simulink model "EthernetDrone"  (Simulink 8.5)
settings: Solver=ode45  StartTime=0.0  StopTime=300  RelTol=abstol/10  AbsTol=abstol
undefined symbols (not defined in the file or in its folder): A, a_noise_seed, a_noise_var, Cd, enu2ecef, g, GPS_DT, h_noise_seed, h_noise_var, I, I_motor, IMU_DT, m, mag_bias, MAG_DT, mag_noise_seed, mag_noise_var, MaxPropRate, MaxPwmWidth, mean_a_bias, mean_w_bias, MinPwmWidth, q0, r0, r1, r2, r3, r4, r_gps, RateToForce, Re, rho, v0, v_noise_seed, v_noise_var, w0, w_noise_seed, w_noise_var
libraries: simulink x7, instrumentlib x4
settings Model: Creator=Mike  LastModifiedBy=Walker  CovSFcnEnable=off
settings SolverCC: ZeroCrossControl=DisableAll
settings DebuggingCC: SolverPrmCheckMsg=warning  FcnCallInpInsideContextMsg=UseLocalSettings

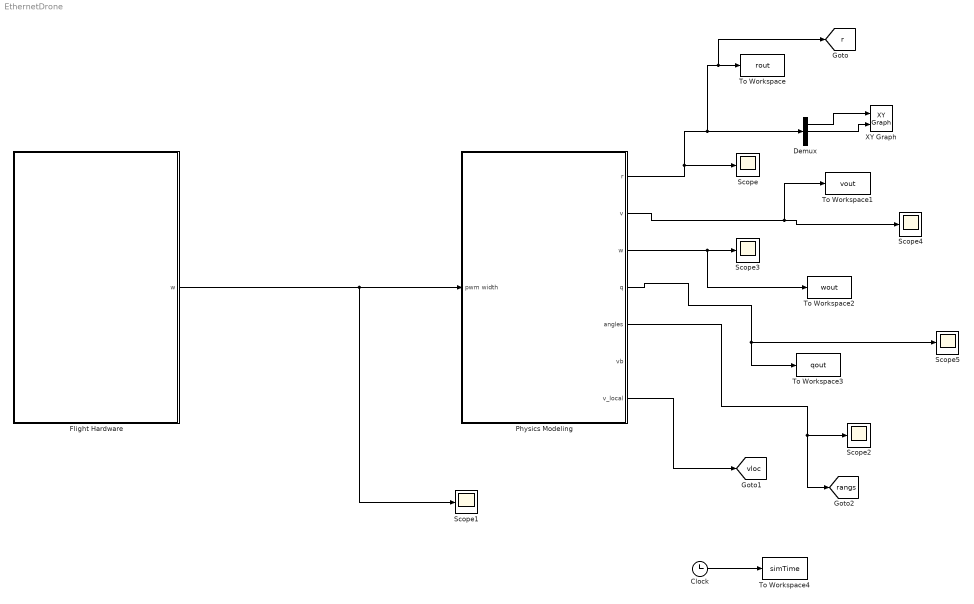
== system EthernetDrone ==
  Clock : Clock
  Demux : Demux  Outputs=3
  Flight Hardware : Subsystem
  Physics Modeling : Subsystem
  Scope{,1..5} (6 alike) : Scope
      Scope settings: TimeRange=100  YMin=4  YMax=17
      Scope1 settings: TimeRange=10  YMin=1.368  YMax=1.3696
      Scope2 settings: TimeRange=300  YMin=-4.5  YMax=4.5  SaveName=ScopeData5
      Scope3 settings: TimeRange=30  YMin=-0.05  YMax=0.05  SaveName=ScopeData13
      Scope4 settings: TimeRange=100  YMin=-4  YMax=8  SaveName=ScopeData38
      Scope5 settings: TimeRange=100  YMin=-0.2  YMax=1  SaveName=ScopeData96
  To Workspace : ToWorkspace  VariableName=rout  SampleTime=IMU_DT
  To Workspace1 : ToWorkspace  VariableName=vout  SampleTime=IMU_DT
  To Workspace2 : ToWorkspace  VariableName=wout  SampleTime=IMU_DT
  To Workspace3 : ToWorkspace  VariableName=qout  SampleTime=IMU_DT
  To Workspace4 : ToWorkspace  VariableName=simTime  SampleTime=IMU_DT
  XY Graph : simulink/Sinks/XY Graph  xmin=-20  xmax=20  ymin=-20  ymax=20  st=1
  tag scope: r=global, rangs=global, vloc=global
  wires:
  Flight Hardware/1(w) -> Physics Modeling/1("pwm width "), Scope1/1
  Physics Modeling/1(r) -> Demux/1, To Workspace/1, [r], Scope/1
  Physics Modeling/5(angles) -> Scope2/1, [rangs]
  Physics Modeling/3(w) -> Scope3/1, To Workspace2/1
  Physics Modeling/2(v) -> Scope4/1, To Workspace1/1
  Demux/1 -> XY Graph/1
  Demux/2 -> XY Graph/2
  Physics Modeling/4(q) -> To Workspace3/1, Scope5/1
  Physics Modeling/7(v_local) -> [vloc]
  Clock/1 -> To Workspace4/1

== system EthernetDrone/Flight Hardware ==
  Sensor Model : Subsystem
  Subsystem : Subsystem
  Subsystem1 : Subsystem
  Subsystem2 : Subsystem
  Subsystem3 : Subsystem
  w : Outport
  wires:
  Sensor Model/2(w_b) -> Subsystem/2(win)
  Sensor Model/1(a_b) -> Subsystem/1(ain)
  Sensor Model/3(h) -> Subsystem1/1(gps)
  Sensor Model/4(mag) -> Subsystem2/1(mag)
  Subsystem3/1(w) -> w/1

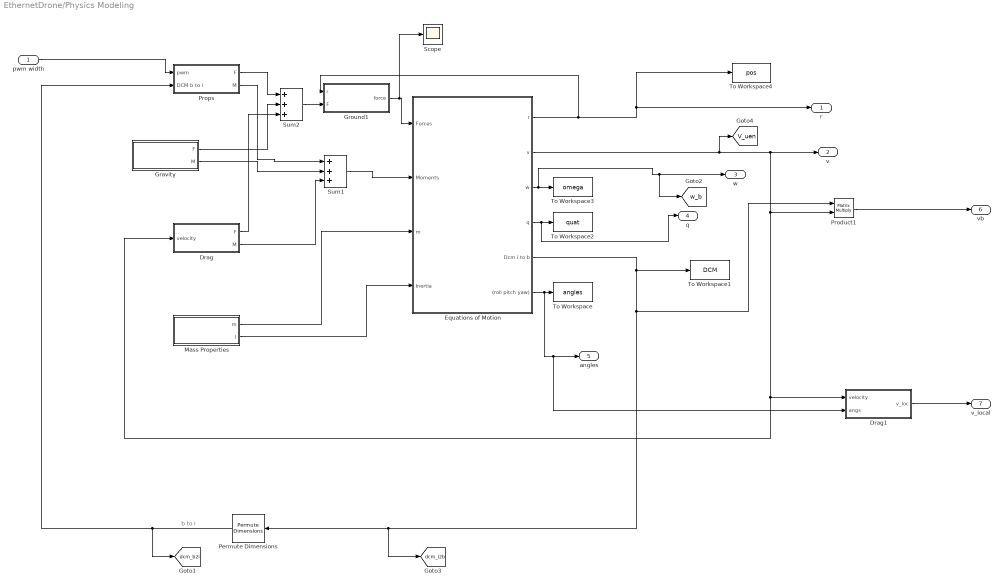
== system EthernetDrone/Physics Modeling ==
  note: b to i
  "pwm width " : Inport
  Drag : Subsystem
  Drag1 : Subsystem
  Equations of Motion : Subsystem
  Gravity : Subsystem
  Ground1 : Subsystem
  Mass Properties : Subsystem
  Permute Dimensions : PermuteDimensions
  Product1 : Product  Multiplication=Matrix(*)  RndMeth=Zero
  Props : Subsystem
  Scope : Scope
      settings: TimeRange=5.350553505535055  YMin=-4  SaveName=ScopeData58
  Sum1 : Sum  Inputs=+++
  Sum2 : Sum  Inputs=+++
  To Workspace : ToWorkspace  VariableName=angles  SampleTime=-1
  To Workspace1 : ToWorkspace  VariableName=DCM  SampleTime=-1
  To Workspace2 : ToWorkspace  VariableName=quat  SampleTime=-1
  To Workspace3 : ToWorkspace  VariableName=omega  SampleTime=-1
  To Workspace4 : ToWorkspace  VariableName=pos  SampleTime=-1
  r : Outport
  v : Outport  Port=2
  w : Outport  Port=3
  q : Outport  Port=4
  angles : Outport  Port=5
  vb : Outport  Port=6
  v_local : Outport  Port=7
  tag scope: V_uen=global, dcm_b2i=global, dcm_i2b=global, w_b=global
  wires:
  Props/1(F) -> Sum2/1
  Gravity/1(F) -> Sum2/2
  Drag/1(F) -> Sum2/3
  Props/2(M) -> Sum1/1
  Gravity/2(M) -> Sum1/2
  Drag/2(M) -> Sum1/3
  Sum1/1 -> Equations of Motion/2(Moments)
  Mass Properties/1(m) -> Equations of Motion/3(m)
  Mass Properties/2(I) -> Equations of Motion/4(Inertia)
  "pwm width "/1 -> Props/1(pwm)
  Equations of Motion/2(v) -> Drag/1(velocity), Drag1/1(velocity), Product1/2, v/1, [V_uen]
  Equations of Motion/1(r) -> Ground1/1(r), To Workspace4/1, r/1
  Equations of Motion/6((roll pitch yaw)) -> To Workspace/1, angles/1, Drag1/2(angs)
  Equations of Motion/5(Dcm i to b) -> To Workspace1/1, Product1/1, Permute Dimensions/1, [dcm_i2b]
  Equations of Motion/4(q) -> To Workspace2/1, q/1
  Equations of Motion/3(w) -> To Workspace3/1, w/1, [w_b]
  Permute Dimensions/1 -> [dcm_b2i], Props/2("DCM b to i ")
  Product1/1 -> vb/1
  Drag1/1(v_loc) -> v_local/1
  Ground1/1(force) -> Scope/1, Equations of Motion/1(Forces)
  Sum2/1 -> Ground1/2(F)

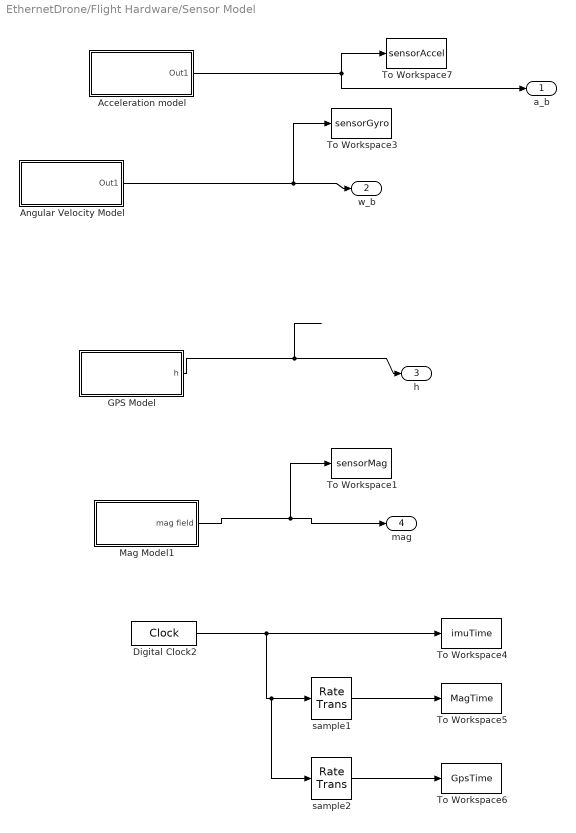
== system EthernetDrone/Flight Hardware/Sensor Model ==
  Acceleration model : Subsystem
  Angular Velocity Model : Subsystem
  Digital Clock2 : DigitalClock  SampleTime=IMU_DT
  GPS Model : Subsystem
  Mag Model1 : Subsystem
  To Workspace1 : ToWorkspace  VariableName=sensorMag  SampleTime=-1
  To Workspace3 : ToWorkspace  VariableName=sensorGyro  SampleTime=-1
  To Workspace4 : ToWorkspace  VariableName=imuTime  SampleTime=-1
  To Workspace5 : ToWorkspace  VariableName=MagTime  SampleTime=-1
  To Workspace6 : ToWorkspace  VariableName=GpsTime  SampleTime=-1
  To Workspace7 : ToWorkspace  VariableName=sensorAccel  SampleTime=-1
  sample1 : RateTransition  OutPortSampleTime=MAG_DT
  sample2 : RateTransition  OutPortSampleTime=GPS_DT
  a_b : Outport
  w_b : Outport  Port=2
  h : Outport  Port=3
  mag : Outport  Port=4
  wires:
  Acceleration model/1(Out1) -> a_b/1, To Workspace7/1
  Angular Velocity Model/1(Out1) -> To Workspace3/1, w_b/1
  GPS Model/1(h) -> h/1
  Mag Model1/1(mag field) -> To Workspace1/1, mag/1
  Digital Clock2/1 -> To Workspace4/1, sample1/1, sample2/1
  sample1/1 -> To Workspace5/1
  sample2/1 -> To Workspace6/1

== system EthernetDrone/Flight Hardware/Subsystem ==
  ain : Inport
  win : Inport  Port=2
  Digital Clock : DigitalClock  SampleTime=IMU_DT
  Mux : Mux  Inputs=3
  UDP Send : instrumentlib/UDP Send  Host=127.0.0.1  Port=8000  LocalPort=-1  EnableBlockingMode=on  ByteOrder=LittleEndian
  wires:
  ain/1 -> Mux/1
  win/1 -> Mux/2
  Digital Clock/1 -> Mux/3
  Mux/1 -> UDP Send/1

== system EthernetDrone/Flight Hardware/Subsystem1 ==
  gps : Inport
  Digital Clock : DigitalClock  SampleTime=GPS_DT
  Mux : Mux  Inputs=2
  UDP Send : instrumentlib/UDP Send  Host=127.0.0.1  Port=8100  LocalPort=-1  EnableBlockingMode=on  ByteOrder=LittleEndian
  wires:
  gps/1 -> Mux/1
  Digital Clock/1 -> Mux/2
  Mux/1 -> UDP Send/1

== system EthernetDrone/Flight Hardware/Subsystem2 ==
  mag : Inport
  Digital Clock : DigitalClock  SampleTime=MAG_DT
  Mux : Mux  Inputs=2
  UDP Send : instrumentlib/UDP Send  Host=127.0.0.1  Port=8200  LocalPort=-1  EnableBlockingMode=on  ByteOrder=LittleEndian
  wires:
  mag/1 -> Mux/1
  Digital Clock/1 -> Mux/2
  Mux/1 -> UDP Send/1

== system EthernetDrone/Flight Hardware/Subsystem3 ==
  Data Type Conversion : DataTypeConversion  OutDataTypeStr=double  SampleTime=IMU_DT
  UDP Receive : instrumentlib/UDP Receive  Host=127.0.0.1  Port=8300  LocalPort=8300  DataSize=4  EnableBlockingMode=on  Timeout=10  SampleTime=-1  DataType=double  ByteOrder=LittleEndian
  w : Outport
  wires:
  UDP Receive/1 -> Data Type Conversion/1
  Data Type Conversion/1 -> w/1

== system EthernetDrone/Physics Modeling/Drag ==
  velocity : Inport
  Abs : Abs
  Constant : Constant  Value=rho*Cd*A
  Gain : Gain  Gain=-0.5
  Product : Product  Inputs=***  RndMeth=Zero
  Scope : Scope
      settings: TimeRange=80  SaveName=ScopeData54
  assume cp = cm : Constant  Value=0
  F : Outport
  M : Outport  Port=2
  tag scope: faero_i=global
  wires:
  velocity/1 -> Abs/1, Gain/1
  Gain/1 -> Product/2
  Abs/1 -> Product/1
  Constant/1 -> Product/3
  assume cp = cm/1 -> M/1
  Product/1 -> F/1, [faero_i], Scope/1

== system EthernetDrone/Physics Modeling/Drag1 ==
  velocity : Inport
  angs : Inport  Port=2
  Embedded MATLAB Function : MATLAB Function  TreatAsAtomicUnit=on
  Product : Product  Multiplication=Matrix(*)  RndMeth=Zero
  v_loc : Outport
  wires:
  velocity/1 -> Product/2
  Product/1 -> v_loc/1
  angs/1 -> Embedded MATLAB Function/1(u)
  Embedded MATLAB Function/1(y) -> Product/1

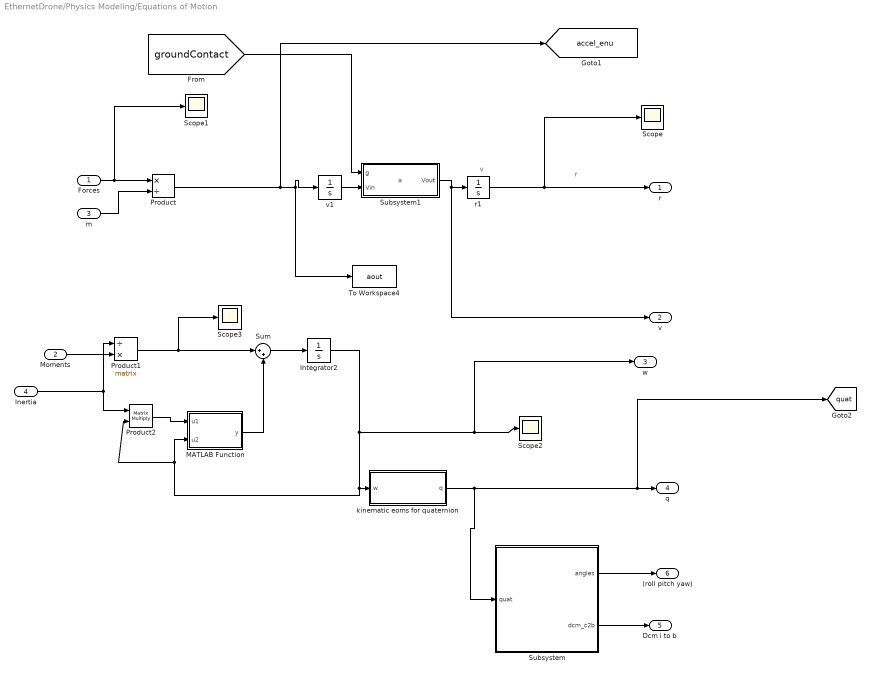
== system EthernetDrone/Physics Modeling/Equations of Motion ==
  note: a
  note: v
  note: r
  Forces : Inport
  Moments : Inport  Port=2
  m : Inport  Port=3
  Inertia : Inport  Port=4
  Integrator2 : Integrator  InitialCondition=w0  AbsoluteTolerance=abstol
  MATLAB Function : MATLAB Function  TreatAsAtomicUnit=on
  Product : Product  Inputs=*/  RndMeth=Zero
  Product1 : Product  Inputs=/*  Multiplication=Matrix(*)  RndMeth=Zero
  Product2 : Product  Inputs=**  Multiplication=Matrix(*)  RndMeth=Zero
  Scope{,1..3} (4 alike) : Scope
      Scope settings: SaveName=ScopeData55
      Scope1 settings: TimeRange=100  SaveName=ScopeData56
      Scope2 settings: TimeRange=50  YMin=-2000  YMax=0  SaveName=ScopeData14
      Scope3 settings: TimeRange=50  YMin=-2000  YMax=0  SaveName=ScopeData37
  Subsystem : Subsystem
  Subsystem1 : Subsystem
  Sum : Sum  Inputs=|++
  To Workspace4 : ToWorkspace  VariableName=aout  SampleTime=-1
  kinematic eoms for quaternion : Subsystem
  r1 : Integrator  InitialCondition=r0  AbsoluteTolerance=abstol
  v1 : Integrator  InitialCondition=v0  AbsoluteTolerance=abstol
  r : Outport
  v : Outport  Port=2
  w : Outport  Port=3
  q : Outport  Port=4
  Dcm i to b : Outport  Port=5
  (roll pitch yaw) : Outport  Port=6
  tag scope: accel_enu=global, quat=global
  wires:
  r1/1 -> Scope/1, r/1
  Forces/1 -> Product/1, Scope1/1
  m/1 -> Product/2
  kinematic eoms for quaternion/1(q) -> Subsystem/1(quat), q/1, [quat]
  Subsystem/2(dcm_c2b) -> Dcm i to b/1
  Subsystem/1(angles) -> (roll pitch yaw)/1
  Inertia/1 -> Product1/1, Product2/1
  Moments/1 -> Product1/2
  Integrator2/1 -> Scope2/1, w/1, kinematic eoms for quaternion/1(w), MATLAB Function/2(u2), Product2/2
  Product2/1 -> MATLAB Function/1(u1)
  Sum/1 -> Integrator2/1
  Product1/1 -> Sum/1, Scope3/1
  MATLAB Function/1(y) -> Sum/2
  Product/1 -> [accel_enu], v1/1, To Workspace4/1
  Subsystem1/1(Vout) -> v/1, r1/1
  v1/1 -> Subsystem1/2(Vin)
  [groundContact] -> Subsystem1/1(g)

== system EthernetDrone/Physics Modeling/Gravity ==
  Ground1 : Subsystem
  No horizontal : Gain  Gain=m
  Scope : Scope
      settings: SaveName=ScopeData57
  cg=cm in this problem : Constant  Value=0
  mg : Constant  Value=[0;0; -m*g ]
  F : Outport
  M : Outport  Port=2
  wires:
  cg=cm in this problem/1 -> M/1
  mg/1 -> F/1, Scope/1
  Ground1/1(accel) -> No horizontal/1

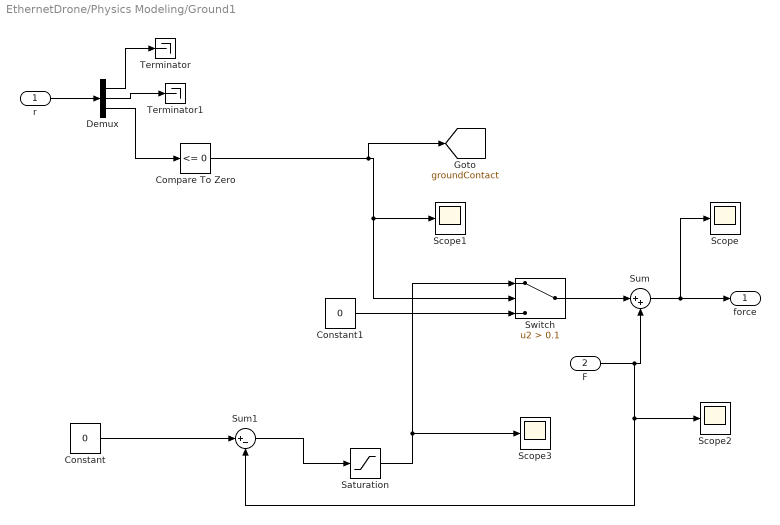
== system EthernetDrone/Physics Modeling/Ground1 ==
  r : Inport
  F : Inport  Port=2
  Compare To Zero : simulink/Logic and Bit Operations/Compare To Zero  relop=<=  OutDataTypeStr=boolean  ZeroCross=off
  Constant : Constant  Value=0
  Constant1 : Constant  Value=0
  Demux : Demux  Outputs=3
  Saturation : Saturate  UpperLimit=inf  LowerLimit=0
  Scope{,1..3} (4 alike) : Scope
      Scope settings: YMin=-10  YMax=10  SaveName=ScopeData88
      Scope1 settings: TimeRange=20  YMin=0.95  YMax=1.05  SaveName=ScopeData51
      Scope2 settings: YMin=-10  YMax=0  SaveName=ScopeData127
      Scope3 settings: YMin=9.5  YMax=20  SaveName=ScopeData128
  Sum : Sum  Inputs=|++
  Sum1 : Sum  Inputs=|+-
  Switch : Switch  Criteria=u2 > Threshold  Threshold=0.1
  Terminator : Terminator
  Terminator1 : Terminator
  force : Outport
  tag scope: groundContact=global
  wires:
  r/1 -> Demux/1
  Demux/1 -> Terminator/1
  Demux/2 -> Terminator1/1
  Demux/3 -> Compare To Zero/1
  Compare To Zero/1 -> [groundContact], Scope1/1, Switch/2
  Saturation/1 -> Switch/1, Scope3/1
  Switch/1 -> Sum/1
  Sum/1 -> Scope/1, force/1
  F/1 -> Scope2/1, Sum1/2, Sum/2
  Constant/1 -> Sum1/1
  Sum1/1 -> Saturation/1
  Constant1/1 -> Switch/3

== system EthernetDrone/Physics Modeling/Mass Properties ==
  Constant : Constant  Value=m
  a : Constant  Value=I
  m : Outport
  I : Outport  Port=2
  tag scope: mass=global
  wires:
  a/1 -> I/1
  Constant/1 -> m/1, [mass]

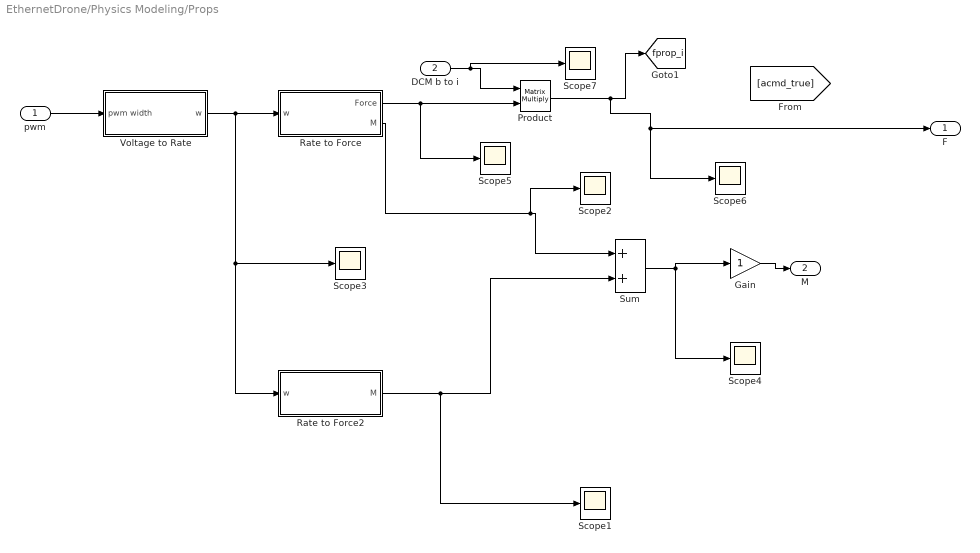
== system EthernetDrone/Physics Modeling/Props ==
  pwm : Inport
  "DCM b to i " : Inport  Port=2
  Gain : Gain
  Product : Product  Multiplication=Matrix(*)  OutDataTypeStr=Inherit: Inherit via back propagation  RndMeth=Nearest
  Rate to Force : Subsystem
  Rate to Force2 : Subsystem
  Scope{1..7} (7 alike) : Scope
      Scope1 settings: TimeRange=50  YMin=0  YMax=200  SaveName=ScopeData2
      Scope2 settings: YMin=-1  YMax=1  SaveName=ScopeData3
      Scope3 settings: TimeRange=50  YMin=-0.2  YMax=0.85  SaveName=ScopeData4
      Scope4 settings: TimeRange=6.110074626865668  YMin=-3.63961038961039e-009  YMax=-3.405844155844153e-009  SaveName=ScopeData11
      Scope5 settings: TimeRange=50  YMin=0  YMax=4e+14  SaveName=ScopeData9
      Scope6 settings: TimeRange=50  YMin=0  YMax=40  SaveName=ScopeData59
      Scope7 settings: TimeRange=0.2158273381295004  YMin=-1  YMax=1  SaveName=ScopeData62
  Sum : Sum
  Voltage to Rate : Subsystem
  F : Outport
  M : Outport  Port=2
  tag scope: fprop_i=global
  wires:
  pwm/1 -> Voltage to Rate/1(pwm width)
  Voltage to Rate/1(w) -> Rate to Force/1(w), Rate to Force2/1(w), Scope3/1
  Sum/1 -> Scope4/1, Gain/1
  Rate to Force/2(M) -> Sum/1, Scope2/1
  Rate to Force2/1(M) -> Sum/2, Scope1/1
  Product/1 -> [fprop_i], Scope6/1, F/1
  "DCM b to i "/1 -> Product/1, Scope7/1
  Rate to Force/1(Force) -> Product/2, Scope5/1
  Gain/1 -> M/1

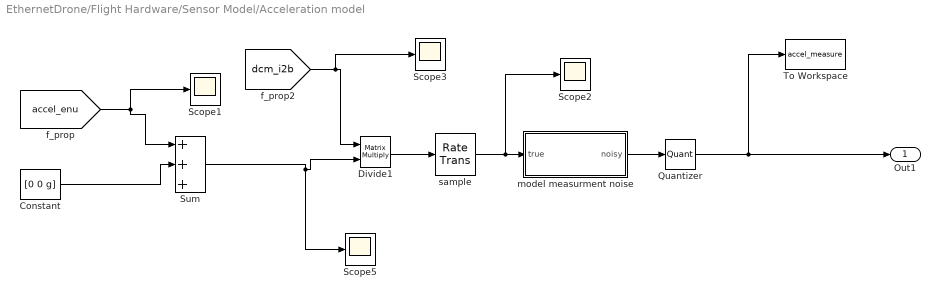
== system EthernetDrone/Flight Hardware/Sensor Model/Acceleration model ==
  Constant : Constant  Value=[0 0 g]
  Divide1 : Product  Inputs=**  Multiplication=Matrix(*)
  Quantizer : Quantizer  QuantizationInterval=AccelQuant
  Scope{1..3,5} (4 alike) : Scope
      Scope1 settings: TimeRange=30  YMin=-50  YMax=50  SaveName=ScopeData46
      Scope2 settings: TimeRange=35  YMin=-2.5  YMax=40  SaveName=ScopeData47
      Scope3 settings: TimeRange=35  YMin=0  YMax=1  SaveName=ScopeData100
      Scope5 settings: TimeRange=49.99000000000001  YMin=9.763194444444443  YMax=9.821527777777776  SaveName=ScopeData101
  Sum : Sum  Inputs=+++
  To Workspace : ToWorkspace  VariableName=accel_measure  SampleTime=-1
  model measurment noise : Subsystem
  sample : RateTransition  X0=[0 0 g]  OutPortSampleTime=IMU_DT
  Out1 : Outport
  wires:
  Constant/1 -> Sum/2
  [accel_enu] -> Sum/1, Scope1/1
  sample/1 -> model measurment noise/1("true "), Scope2/1
  Divide1/1 -> sample/1
  Sum/1 -> Divide1/2, Scope5/1
  [dcm_i2b] -> Divide1/1, Scope3/1
  model measurment noise/1(noisy) -> Quantizer/1
  Quantizer/1 -> To Workspace/1, Out1/1

== system EthernetDrone/Flight Hardware/Sensor Model/Angular Velocity Model ==
  Product : Product  Multiplication=Matrix(*)  RndMeth=Zero
  Quantizer : Quantizer  QuantizationInterval=GyroQuant
  Scope : Scope
      settings: TimeRange=30  YMin=-0.06  YMax=0.08  SaveName=ScopeData61
  Sum : Sum  Inputs=|++
  To Workspace1 : ToWorkspace  VariableName=omega_measure  SampleTime=-1
  earth rot rate (rads/sec)--assume at lat,log h (0,0,0) : Constant  Value=[0;0;0.00007272205]
  model measurment noise : Subsystem
  sample : RateTransition  OutPortSampleTime=IMU_DT
  Out1 : Outport
  wires:
  sample/1 -> model measurment noise/1("true ")
  earth rot rate (rads/sec)--assume at lat,log h (0,0,0)/1 -> Product/2
  [dcm_i2b] -> Product/1
  Product/1 -> ?
  [w_b] -> Sum/1
  Sum/1 -> sample/1
  model measurment noise/1(noisy) -> Quantizer/1
  Quantizer/1 -> To Workspace1/1, Scope/1, Out1/1

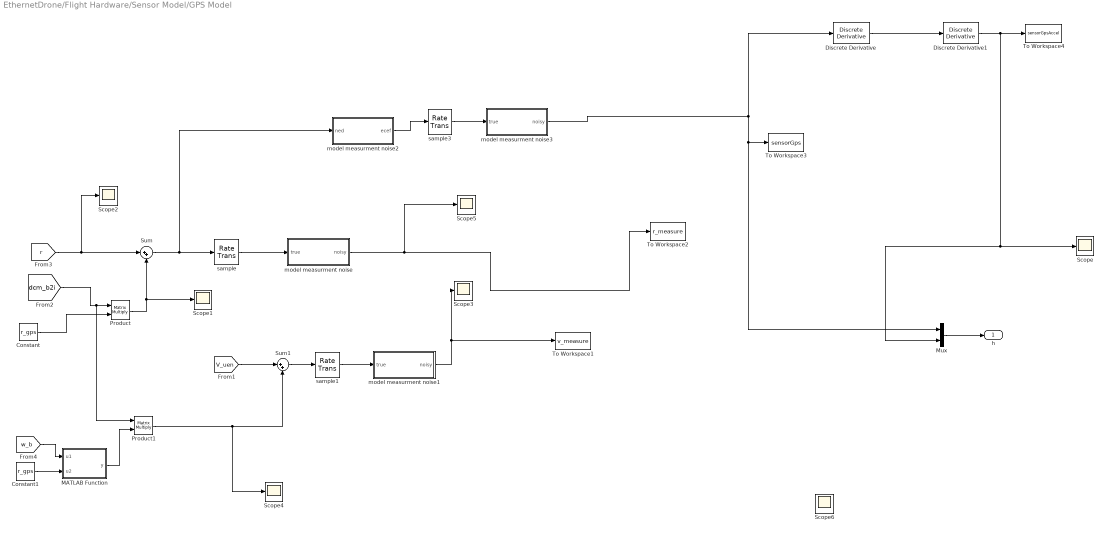
== system EthernetDrone/Flight Hardware/Sensor Model/GPS Model ==
  Constant : Constant  Value=r_gps
  Constant1 : Constant  Value=r_gps
  Discrete Derivative : simulink/Discrete/Discrete Derivative  gainval=1  ICPrevScaledInput=0.0  InputProcessing=Inherited  OutMin=[]  OutMax=[]  OutDataType=fixdt(1, 16)  OutScaling=2^-10  DoSatur=off
  Discrete Derivative1 : simulink/Discrete/Discrete Derivative  gainval=1.0  ICPrevScaledInput=0  InputProcessing=Inherited  OutMin=[]  OutMax=[]  OutDataType=fixdt(1, 16)  OutScaling=2^-10  DoSatur=off
  MATLAB Function : MATLAB Function  TreatAsAtomicUnit=on
  Mux : Mux  Inputs=2
  Product : Product  Multiplication=Matrix(*)  RndMeth=Zero
  Product1 : Product  Multiplication=Matrix(*)  RndMeth=Zero
  Scope{,1..6} (7 alike) : Scope
      Scope settings: SaveName=ScopeData49
      Scope1 settings: TimeRange=30  YMin=-1  YMax=1  SaveName=ScopeData98
      Scope2 settings: TimeRange=30  YMin=1  YMax=5.25  SaveName=ScopeData97
      Scope3 settings: TimeRange=30  YMin=-0.075  YMax=0.2  SaveName=ScopeData103
      Scope4 settings: TimeRange=30  YMin=-0.35  YMax=0.125  SaveName=ScopeData104
      Scope5 settings: TimeRange=30  YMin=3.5  YMax=11  SaveName=ScopeData94
      Scope6 settings: TimeRange=10  YMin=0.95  YMax=1.05  SaveName=ScopeData102
  Sum : Sum  Inputs=|++
  Sum1 : Sum  Inputs=|++
  To Workspace1 : ToWorkspace  VariableName=v_measure  SampleTime=GPS_DT
  To Workspace2 : ToWorkspace  VariableName=r_measure  SampleTime=IMU_DT
  To Workspace3 : ToWorkspace  VariableName=sensorGps  SampleTime=-1
  To Workspace4 : ToWorkspace  VariableName=sensorGpsAccel  SampleTime=IMU_DT
  model measurment noise : Subsystem
  model measurment noise1 : Subsystem
  model measurment noise2 : Subsystem
  model measurment noise3 : Subsystem
  sample : RateTransition  OutPortSampleTime=GPS_DT
  sample1 : RateTransition  OutPortSampleTime=GPS_DT
  sample3 : RateTransition  OutPortSampleTime=GPS_DT
  h : Outport  OutDataTypeStr=double
  wires:
  sample/1 -> model measurment noise/1("true ")
  sample1/1 -> model measurment noise1/1("true ")
  model measurment noise1/1(noisy) -> Scope3/1, To Workspace1/1
  Constant/1 -> Product/2
  [dcm_b2i] -> Product/1, Product1/1
  Sum/1 -> model measurment noise2/1("ned "), sample/1
  Product/1 -> Sum/2, Scope1/1
  [r] -> Sum/1, Scope2/1
  Sum1/1 -> sample1/1
  [V_uen] -> Sum1/1
  Constant1/1 -> MATLAB Function/2(u2)
  [w_b] -> MATLAB Function/1(u1)
  Product1/1 -> Sum1/2, Scope4/1
  MATLAB Function/1(y) -> Product1/2
  ? -> ?
  model measurment noise2/1(ecef) -> sample3/1
  sample3/1 -> model measurment noise3/1("true ")
  model measurment noise3/1(noisy) -> Discrete Derivative/1, To Workspace3/1, Mux/1
  model measurment noise/1(noisy) -> Scope5/1, To Workspace2/1
  Discrete Derivative/1 -> Discrete Derivative1/1
  Discrete Derivative1/1 -> Scope/1, Mux/2, To Workspace4/1
  Mux/1 -> h/1

== system EthernetDrone/Flight Hardware/Sensor Model/Mag Model1 ==
  Embedded MATLAB Function : MATLAB Function  TreatAsAtomicUnit=on
  Product : Product  Multiplication=Matrix(*)  RndMeth=Zero
  Scope4 : Scope
      settings: TimeRange=300  YMin=-0.8  YMax=0.05  SaveName=ScopeData108
  To Workspace3 : ToWorkspace  VariableName=mag_measure  SampleTime=MAG_DT
  model measurment noise1 : Subsystem
  sample1 : RateTransition  OutPortSampleTime=MAG_DT
  mag field : Outport  OutDataTypeStr=double
  wires:
  sample1/1 -> model measurment noise1/1("true ")
  Embedded MATLAB Function/1(Mhat) -> Product/2
  [dcm_i2b] -> Product/1
  model measurment noise1/1(noisy) -> Scope4/1, mag field/1, To Workspace3/1
  Product/1 -> sample1/1

== system EthernetDrone/Physics Modeling/Equations of Motion/Subsystem ==
  note: Based on Prof Howell AAE 440 Notes
  note: C is row notation so transpose it!
  quat : Inport
  Permute Dimensions : PermuteDimensions
  solve direction cosine matrix : Subsystem
  angles : Outport
  dcm_c2b : Outport  Port=2
  wires:
  quat/1 -> solve direction cosine matrix/1(quat)
  solve direction cosine matrix/2(roll pitch yaw) -> angles/1
  solve direction cosine matrix/1(C) -> Permute Dimensions/1
  Permute Dimensions/1 -> dcm_c2b/1

== system EthernetDrone/Physics Modeling/Equations of Motion/Subsystem1 ==
  g : Inport
  Vin : Inport  Port=2
  Saturation : Saturate  UpperLimit=[0 0 inf]  LowerLimit=[0 0 0]
  Switch : Switch  Criteria=u2 > Threshold
  Vout : Outport
  wires:
  Switch/1 -> Vout/1
  Vin/1 -> Saturation/1, Switch/3
  g/1 -> Switch/2
  Saturation/1 -> Switch/1

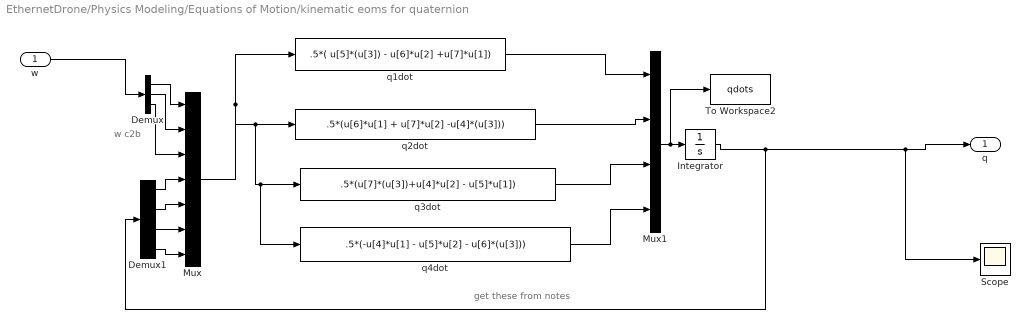
== system EthernetDrone/Physics Modeling/Equations of Motion/kinematic eoms for quaternion ==
  note: get these from notes
  note: w c2b
  w : Inport
  Demux : Demux  Outputs=3
  Demux1 : Demux
  Integrator : Integrator  InitialCondition=q0  AbsoluteTolerance=abstol  IgnoreLimit=on
  Mux : Mux  Inputs=7
  Mux1 : Mux
  Scope : Scope
      settings: SaveName=ScopeData60
  To Workspace2 : ToWorkspace  VariableName=qdots  SampleTime=-1
  q1dot : Fcn  Expr=.5*( u[5]*(u[3]) - u[6]*u[2] +u[7]*u[1])
  q2dot : Fcn  Expr=.5*(u[6]*u[1] + u[7]*u[2] -u[4]*(u[3]))
  q3dot : Fcn  Expr=.5*(u[7]*(u[3])+u[4]*u[2] - u[5]*u[1])
  q4dot : Fcn  Expr=.5*(-u[4]*u[1] - u[5]*u[2] - u[6]*(u[3]))
  q : Outport
  wires:
  Mux1/1 -> Integrator/1, To Workspace2/1
  Integrator/1 -> Demux1/1, q/1, Scope/1
  q4dot/1 -> Mux1/4
  q3dot/1 -> Mux1/3
  q2dot/1 -> Mux1/2
  q1dot/1 -> Mux1/1
  Mux/1 -> q1dot/1, q2dot/1, q3dot/1, q4dot/1
  w/1 -> Demux/1
  Demux/1 -> Mux/1
  Demux/2 -> Mux/2
  Demux/3 -> Mux/3
  Demux1/1 -> Mux/4
  Demux1/2 -> Mux/5
  Demux1/3 -> Mux/6
  Demux1/4 -> Mux/7

== system EthernetDrone/Physics Modeling/Gravity/Ground1 ==
  r : Inport
  G : Inport  Port=2
  Compare To Zero : simulink/Logic and Bit Operations/Compare To Zero  relop=<=  OutDataTypeStr=boolean  ZeroCross=off
  Demux : Demux  Outputs=3
  No horizontal : Gain  Gain=[0 0 1]
  Saturation : Saturate  UpperLimit=[0 0 inf]  LowerLimit=[0 0 0]
  Scope : Scope
      settings: YMin=-0.0014  YMax=0  SaveName=ScopeData88
  Scope1 : Scope
      settings: TimeRange=20  YMin=0  YMax=3e-14  SaveName=ScopeData51
  Switch : Switch  Criteria=u2 > Threshold  Threshold=0.1
  Terminator : Terminator
  Terminator1 : Terminator
  accel : Outport
  wires:
  r/1 -> Demux/1
  Demux/1 -> Terminator/1
  Demux/2 -> Terminator1/1
  Demux/3 -> Compare To Zero/1
  G/1 -> No horizontal/1, Scope1/1, Switch/3
  Compare To Zero/1 -> Switch/2
  Switch/1 -> Scope/1, accel/1
  No horizontal/1 -> Saturation/1
  Saturation/1 -> Switch/1

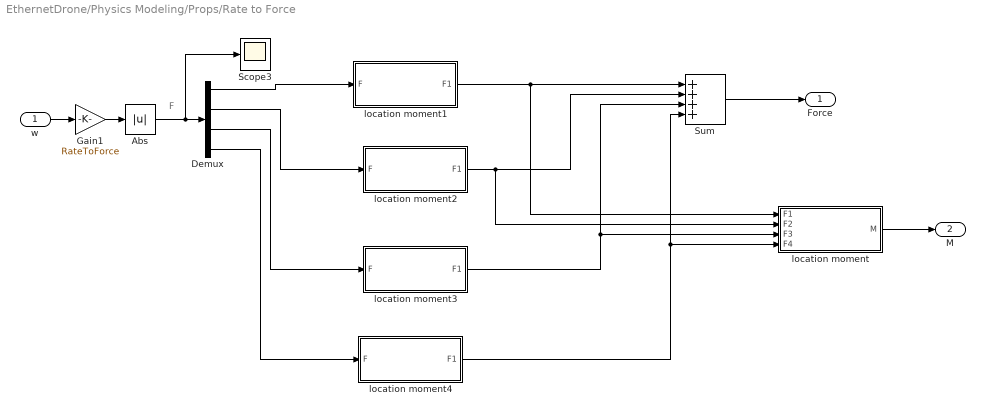
== system EthernetDrone/Physics Modeling/Props/Rate to Force ==
  note: F
  w : Inport
  Abs : Abs
  Demux : Demux
  Gain1 : Gain  Gain=RateToForce
  Scope3 : Scope
      settings: TimeRange=50  YMin=2.32987  YMax=2.57513  SaveName=ScopeData8
  Sum : Sum  Inputs=++++
  location moment : Subsystem
  location moment1 : Subsystem
  location moment2 : Subsystem
  location moment3 : Subsystem
  location moment4 : Subsystem
  Force : Outport
  M : Outport  Port=2
  wires:
  location moment/1(M) -> M/1
  Sum/1 -> Force/1
  location moment1/1(F1) -> Sum/1, location moment/1(F1)
  location moment2/1(F1) -> Sum/2, location moment/2(F2)
  location moment3/1(F1) -> Sum/3, location moment/3(F3)
  location moment4/1(F1) -> Sum/4, location moment/4(F4)
  Demux/1 -> location moment1/1(F)
  Demux/2 -> location moment2/1(F)
  Demux/3 -> location moment3/1(F)
  Demux/4 -> location moment4/1(F)
  Abs/1 -> Demux/1, Scope3/1
  w/1 -> Gain1/1
  Gain1/1 -> Abs/1

== system EthernetDrone/Physics Modeling/Props/Rate to Force2 ==
  w : Inport
  Demux : Demux
  Gain : Gain  Gain=I_motor
  Motor 1 : Subsystem
  Motor 2 : Subsystem
  Motor 3 : Subsystem
  Motor 4 : Subsystem
  Sum : Sum  Inputs=++++
  M : Outport
  wires:
  w/1 -> Gain/1
  Gain/1 -> Demux/1
  Demux/1 -> Motor 1/1(w1)
  Demux/2 -> Motor 2/1(w2)
  Demux/4 -> Motor 4/1(w4)
  Motor 3/1(M) -> Sum/3
  Motor 4/1(M) -> Sum/4
  Motor 2/1(M) -> Sum/2
  Motor 1/1(M) -> Sum/1
  Sum/1 -> M/1
  Demux/3 -> Motor 3/1(w3)

== system EthernetDrone/Physics Modeling/Props/Voltage to Rate ==
  pwm width : Inport
  Constant : Constant  Value=MinPwmWidth
  Gain : Gain  Gain=1/(MaxPwmWidth - MinPwmWidth)
  Gain1 : Gain  Gain=MaxPropRate
  Rotation Direction : Gain  Gain=[1 -1 1 -1]
  Sum : Sum  Inputs=|+-
  w : Outport
  wires:
  Constant/1 -> Sum/2
  Sum/1 -> Gain/1
  Rotation Direction/1 -> w/1
  pwm width/1 -> Sum/1
  Gain1/1 -> Rotation Direction/1
  Gain/1 -> Gain1/1

== system EthernetDrone/Flight Hardware/Sensor Model/Acceleration model/model measurment noise ==
  "true " : Inport
  Random Number : RandomNumber  Mean=mean_a_bias  Variance=a_noise_var  Seed=a_noise_seed  SampleTime=IMU_DT
  Scope : Scope
      settings: TimeRange=30  YMin=-0.3  YMax=0.4  SaveName=ScopeData44
  Sum : Sum  Inputs=|++
  noisy : Outport
  wires:
  Random Number/1 -> Scope/1, Sum/2
  "true "/1 -> Sum/1
  Sum/1 -> noisy/1

== system EthernetDrone/Flight Hardware/Sensor Model/Angular Velocity Model/model measurment noise ==
  "true " : Inport
  Random Number : RandomNumber  Mean=mean_w_bias  Variance=w_noise_var  Seed=w_noise_seed  SampleTime=IMU_DT
  Scope : Scope
      settings: TimeRange=60  YMin=-0.4  YMax=0.45  SaveName=ScopeData43
  Sum : Sum  Inputs=|++
  noisy : Outport
  wires:
  Random Number/1 -> Scope/1, Sum/2
  "true "/1 -> Sum/1
  Sum/1 -> noisy/1

== system EthernetDrone/Flight Hardware/Sensor Model/GPS Model/model measurment noise ==
  "true " : Inport
  Discrete Derivative : simulink/Discrete/Discrete Derivative  gainval=1  ICPrevScaledInput=0.0  InputProcessing=Inherited  OutMin=[]  OutMax=[]  OutDataType=fixdt(1, 16)  OutScaling=2^-10  DoSatur=off
  Discrete Derivative1 : simulink/Discrete/Discrete Derivative  gainval=1.0  ICPrevScaledInput=0  InputProcessing=Inherited  OutMin=[]  OutMax=[]  OutDataType=fixdt(1, 16)  OutScaling=2^-10  DoSatur=off
  Random Number : RandomNumber  Variance=h_noise_var  Seed=h_noise_seed  SampleTime=GPS_DT
  Scope{,3..4,6} (4 alike) : Scope
      Scope settings: YMin=-0.15  YMax=0.15  SaveName=ScopeData43
      Scope3 settings: TimeRange=50  YMin=-12.5  YMax=12.5  SaveName=ScopeData73
      Scope4 settings: TimeRange=50  SaveName=ScopeData123
      Scope6 settings: TimeRange=10  YMin=-12.5  YMax=12.5  SaveName=ScopeData124
  Sum : Sum  Inputs=|++  AccumDataTypeStr=double
  noisy : Outport
  wires:
  "true "/1 -> Sum/1
  Sum/1 -> noisy/1
  Random Number/1 -> Discrete Derivative/1, Scope3/1, Scope/1, Sum/2
  Discrete Derivative/1 -> Scope6/1, Discrete Derivative1/1
  Discrete Derivative1/1 -> Scope4/1

== system EthernetDrone/Flight Hardware/Sensor Model/GPS Model/model measurment noise1 ==
  "true " : Inport
  Random Number : RandomNumber  Variance=v_noise_var  Seed=v_noise_seed  SampleTime=GPS_DT
  Scope : Scope
      settings: SaveName=ScopeData43
  Sum : Sum  Inputs=|++  AccumDataTypeStr=double  OutDataTypeStr=Inherit: Same as first input
  noisy : Outport
  wires:
  Random Number/1 -> Scope/1, Sum/2
  "true "/1 -> Sum/1
  Sum/1 -> noisy/1

== system EthernetDrone/Flight Hardware/Sensor Model/GPS Model/model measurment noise2 ==
  "ned " : Inport
  Constant : Constant  Value=enu2ecef
  Constant1 : Constant  Value=[0;0;Re]
  Divide : Product  Inputs=**  Multiplication=Matrix(*)
  Sum : Sum  Inputs=|++
  ecef : Outport
  wires:
  Constant/1 -> Divide/1
  Constant1/1 -> Sum/2
  "ned "/1 -> Sum/1
  Sum/1 -> Divide/2
  Divide/1 -> ecef/1

== system EthernetDrone/Flight Hardware/Sensor Model/GPS Model/model measurment noise3 ==
  "true " : Inport
  Random Number : RandomNumber  Variance=h_noise_var  Seed=h_noise_seed  SampleTime=GPS_DT
  Scope : Scope
      settings: SaveName=ScopeData43
  Sum : Sum  Inputs=|++  AccumDataTypeStr=double
  noisy : Outport
  wires:
  Random Number/1 -> Scope/1, Sum/2
  "true "/1 -> Sum/1
  Sum/1 -> noisy/1

== system EthernetDrone/Flight Hardware/Sensor Model/Mag Model1/model measurment noise1 ==
  "true " : Inport
  Random Number : RandomNumber  Mean=mag_bias  Variance=mag_noise_var  Seed=mag_noise_seed  SampleTime=MAG_DT
  Scope : Scope
      settings: TimeRange=300  SaveName=ScopeData43
  Sum : Sum  Inputs=|++
  noisy : Outport
  wires:
  Random Number/1 -> Scope/1, Sum/2
  "true "/1 -> Sum/1
  Sum/1 -> noisy/1

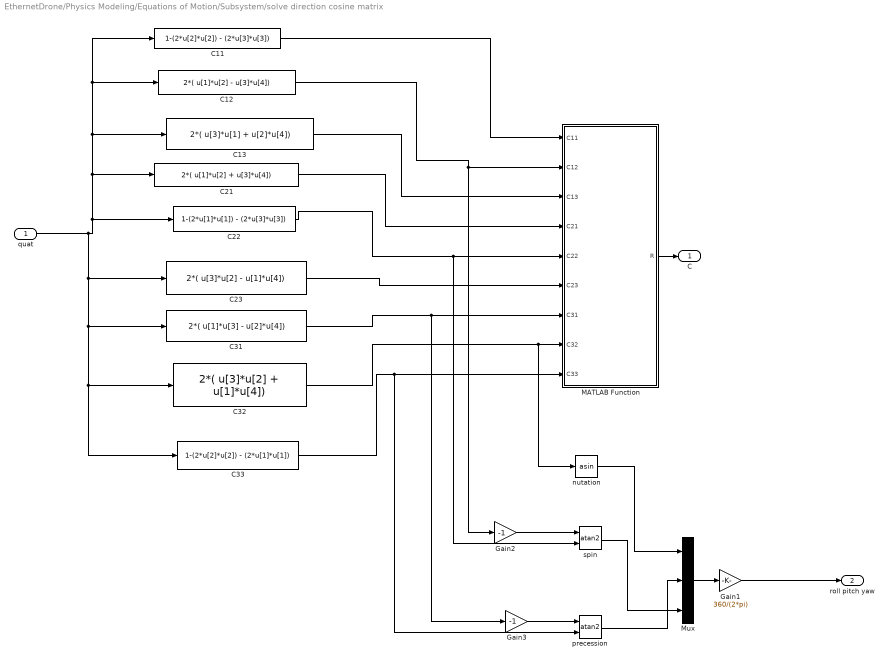
== system EthernetDrone/Physics Modeling/Equations of Motion/Subsystem/solve direction cosine matrix ==
  quat : Inport
  C11 : Fcn  Expr=1-(2*u[2]*u[2]) - (2*u[3]*u[3])
  C12 : Fcn  Expr=2*( u[1]*u[2] - u[3]*u[4])
  C13 : Fcn  Expr=2*( u[3]*u[1] + u[2]*u[4])
  C21 : Fcn  Expr=2*( u[1]*u[2] + u[3]*u[4])
  C22 : Fcn  Expr=1-(2*u[1]*u[1]) - (2*u[3]*u[3])
  C23 : Fcn  Expr=2*( u[3]*u[2] - u[1]*u[4])
  C31 : Fcn  Expr=2*( u[1]*u[3] - u[2]*u[4])
  C32 : Fcn  Expr=2*( u[3]*u[2] + u[1]*u[4])
  C33 : Fcn  Expr=1-(2*u[2]*u[2]) - (2*u[1]*u[1])
  Gain1 : Gain  Gain=360/(2*pi)
  Gain2 : Gain  Gain=-1
  Gain3 : Gain  Gain=-1
  MATLAB Function : MATLAB Function  TreatAsAtomicUnit=on
  Mux : Mux  Inputs=3
  nutation : Trigonometry  Operator=asin
  precession : Trigonometry  Operator=atan2
  spin : Trigonometry  Operator=atan2
  C : Outport
  roll pitch yaw : Outport  Port=2
  wires:
  quat/1 -> C13/1, C11/1, C12/1, C21/1, C22/1, C23/1, C31/1, C33/1, C32/1
  C11/1 -> MATLAB Function/1(C11)
  C12/1 -> MATLAB Function/2(C12), Gain2/1
  C13/1 -> MATLAB Function/3(C13)
  C21/1 -> MATLAB Function/4(C21)
  C22/1 -> MATLAB Function/5(C22), spin/2
  C23/1 -> MATLAB Function/6(C23)
  C31/1 -> MATLAB Function/7(C31), Gain3/1
  C32/1 -> MATLAB Function/8(C32), nutation/1
  C33/1 -> MATLAB Function/9(C33), precession/2
  Gain1/1 -> roll pitch yaw/1
  Mux/1 -> Gain1/1
  Gain2/1 -> spin/1
  Gain3/1 -> precession/1
  nutation/1 -> Mux/1
  spin/1 -> Mux/3
  precession/1 -> Mux/2
  MATLAB Function/1(R) -> C/1

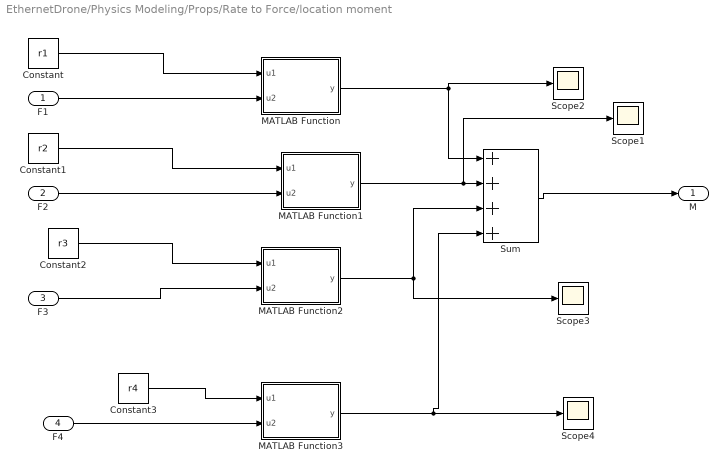
== system EthernetDrone/Physics Modeling/Props/Rate to Force/location moment ==
  F1 : Inport
  F2 : Inport  Port=2
  F3 : Inport  Port=3
  F4 : Inport  Port=4
  Constant : Constant  Value=r1
  Constant1 : Constant  Value=r2
  Constant2 : Constant  Value=r3
  Constant3 : Constant  Value=r4
  MATLAB Function : MATLAB Function  TreatAsAtomicUnit=on
  MATLAB Function1 : MATLAB Function  TreatAsAtomicUnit=on
  MATLAB Function2 : MATLAB Function  TreatAsAtomicUnit=on
  MATLAB Function3 : MATLAB Function  TreatAsAtomicUnit=on
  Scope{1..4} (4 alike) : Scope
      Scope1 settings: YMin=-1  YMax=1  SaveName=ScopeData17
      Scope2 settings: TimeRange=50  YMin=-1  YMax=1  SaveName=ScopeData16
      Scope3 settings: TimeRange=50  YMin=-1  YMax=1  SaveName=ScopeData18
      Scope4 settings: TimeRange=50  YMin=-1  YMax=1  SaveName=ScopeData19
  Sum : Sum  Inputs=++++
  M : Outport
  wires:
  F2/1 -> MATLAB Function1/2(u2)
  F1/1 -> MATLAB Function/2(u2)
  Constant/1 -> MATLAB Function/1(u1)
  Sum/1 -> M/1
  MATLAB Function/1(y) -> Scope2/1, Sum/1
  MATLAB Function1/1(y) -> Sum/2, Scope1/1
  MATLAB Function2/1(y) -> Scope3/1, Sum/3
  MATLAB Function3/1(y) -> Sum/4, Scope4/1
  Constant1/1 -> MATLAB Function1/1(u1)
  Constant2/1 -> MATLAB Function2/1(u1)
  F3/1 -> MATLAB Function2/2(u2)
  F4/1 -> MATLAB Function3/2(u2)
  Constant3/1 -> MATLAB Function3/1(u1)

== system EthernetDrone/Physics Modeling/Props/Rate to Force/location moment1 ==
  F : Inport
  Constant : Constant  Value=0
  Mux : Mux  Inputs=3
  F1 : Outport
  wires:
  Constant/1 -> Mux/2, Mux/1
  F/1 -> Mux/3
  Mux/1 -> F1/1

== system EthernetDrone/Physics Modeling/Props/Rate to Force/location moment2 ==
  F : Inport
  Constant : Constant  Value=0
  Mux : Mux  Inputs=3
  F1 : Outport
  wires:
  Constant/1 -> Mux/2, Mux/1
  F/1 -> Mux/3
  Mux/1 -> F1/1

== system EthernetDrone/Physics Modeling/Props/Rate to Force/location moment3 ==
  F : Inport
  Constant : Constant  Value=0
  Mux : Mux  Inputs=3
  F1 : Outport
  wires:
  Constant/1 -> Mux/2, Mux/1
  F/1 -> Mux/3
  Mux/1 -> F1/1

== system EthernetDrone/Physics Modeling/Props/Rate to Force/location moment4 ==
  F : Inport
  Constant : Constant  Value=0
  Mux : Mux  Inputs=3
  F1 : Outport
  wires:
  Constant/1 -> Mux/2, Mux/1
  F/1 -> Mux/3
  Mux/1 -> F1/1

== system EthernetDrone/Physics Modeling/Props/Rate to Force2/Motor 1 ==
  w1 : Inport
  Constant : Constant  Value=0
  Gain : Gain
  Mux : Mux  Inputs=3
  M : Outport
  wires:
  Mux/1 -> M/1
  Constant/1 -> Mux/2, Mux/1
  Gain/1 -> Mux/3
  w1/1 -> Gain/1

== system EthernetDrone/Physics Modeling/Props/Rate to Force2/Motor 2 ==
  w2 : Inport
  Constant : Constant  Value=0
  Gain : Gain
  Mux : Mux  Inputs=3
  M : Outport
  wires:
  Mux/1 -> M/1
  Constant/1 -> Mux/2, Mux/1
  Gain/1 -> Mux/3
  w2/1 -> Gain/1

== system EthernetDrone/Physics Modeling/Props/Rate to Force2/Motor 3 ==
  w3 : Inport
  Constant : Constant  Value=0
  Gain : Gain
  Mux : Mux  Inputs=3
  M : Outport
  wires:
  Mux/1 -> M/1
  Constant/1 -> Mux/2, Mux/1
  Gain/1 -> Mux/3
  w3/1 -> Gain/1

== system EthernetDrone/Physics Modeling/Props/Rate to Force2/Motor 4 ==
  w4 : Inport
  Constant : Constant  Value=0
  Gain : Gain
  Mux : Mux  Inputs=3
  M : Outport
  wires:
  Mux/1 -> M/1
  Constant/1 -> Mux/2, Mux/1
  Gain/1 -> Mux/3
  w4/1 -> Gain/1

== matlab function Physics Modeling/Drag1/Embedded MATLAB Function ==
  data: u input double; y output double
function y = fcn(u)
%#eml

y = [ cosd(u(3)), sind(u(3)) , 0;  -sind(u(3)), cosd(u(3)) 0 ; 0 , 0 , 1];

== matlab function Physics Modeling/Equations of Motion/MATLAB Function ==
  data: u1 input double; y output double; u2 input double
function y = fcn(u1,u2)
%#codegen

y = cross(u1,u2);

== matlab function Flight Hardware/Sensor Model/GPS Model/MATLAB Function ==
  data: u1 input double; y output double; u2 input double
function y = fcn(u1,u2)
%#codegen

y = cross(u1,u2);

== matlab function Flight Hardware/Sensor Model/Mag Model1/Embedded MATLAB Function ==
  data: Mhat output double
function Mhat  = Calc_Mag_Field
%#eml


colat = 90-32.2;
Bn = -sind(colat);
Bu = -2*cosd(colat);
M = [0 Bn Bu]';

Mhat = M./sqrt(dot(M,M));
Mhat = [0 30.6 -38.7]';

== matlab function Physics Modeling/Equations of Motion/Subsystem/solve direction cosine matrix/MATLAB Function ==
  data: C11 input double; R output double; C12 input double; C13 input double; C21 input double; C22 input double; C23 input double; C31 input double; C32 input double; C33 input double
function R = Create3x3(C11,C12,C13,C21,C22,C23,C31,C32,C33)

R = [ C11,C12,C13; C21,C22,C23 ; C31, C32 , C33];

== matlab function Physics Modeling/Props/Rate to Force/location moment/MATLAB Function ==
  data: u1 input double; y output double; u2 input double
function y = fcn(u1,u2)
%#codegen

y = cross(u1,u2);

== matlab function Physics Modeling/Props/Rate to Force/location moment/MATLAB Function1 ==
  data: u1 input double; y output double; u2 input double
function y = fcn(u1,u2)
%#codegen

y = cross(u1,u2);

== matlab function Physics Modeling/Props/Rate to Force/location moment/MATLAB Function2 ==
  data: u1 input double; y output double; u2 input double
function y = fcn(u1,u2)
%#codegen

y = cross(u1,u2);

== matlab function Physics Modeling/Props/Rate to Force/location moment/MATLAB Function3 ==
  data: u1 input double; y output double; u2 input double
function y = fcn(u1,u2)
%#codegen

y = cross(u1,u2);
